simulink library "Lib_Solve_SSNRSolverJC_TMATS"  (R2015a)
settings: Solver=ode45  StartTime=0.0  StopTime=10.0  RelTol=1e-3
libraries: Lib_NM_JacobianCalc_TMATS x1, Lib_NM_NewtonRaphsonSolver_TMATS x1
Description:
  | Thomas Modules
settings Model: Creator=jwchapm2  LastModifiedBy=jwchapm2
settings OptimizationCC: ExpressionDepthLimit=2147483647
settings DebuggingCC: UnderspecifiedInitializationDetection=Classic  MergeDetectMultiDrivingBlocksExec=none  SolverPrmCheckMsg=warning  StateNameClashWarn=warning

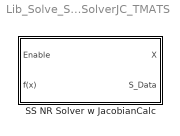
== system Lib_Solve_SSNRSolverJC_TMATS ==
  SS NR Solver w JacobianCalc : Subsystem  mask(T-MATS: SS NR Solver w Jacobian Calc Library Block){SJac_Per_M=[0.01 0.01 0.01;-0.01 -0.01,-0.01], SNR_IC_M=[1; 2; 3], SNR_DX_M=5, SNR_Mx_M=100000, SNR_Mn_M=0.00001, SJacobianAttempts_M=20, Cond_Limits_M=0.0001}
      mask prompts: SJac_Per_M "SJac_Per_M - Jacobian Perturbation size (frac)(nxm)"; SNR_IC_M "SNR_IC_M - Newton Raphson Initial Conditions (mx1)"; SNR_DX_M "SNR_DX_M - Newton Raphson step size limit (%) (1x1)"; SNR_Mx_M "SNR_Mx_M - Newton Raphson max limit (1x1 or mx1)"; SNR_Mn_M "SNR_Mn_M - Newton Raphson min limit (1x1 or mx1)"; SJacobianAttempts_M "SJacobianAttempts_M - Newton Raphson attempts before the Jacobian recalculation (1x1)"; Cond_Limits_M "Cond_Limits_M - Iteration Conditions Limits (mx1 or 1x1)"
      mask help:
      | The Steady State Newton Raphson Solver with Jacobian Calculator block will
      | supply the inputs to iteratively drive the outputs of a system to zero.
      |
      | This will be performed in three steps.
      | 1) Jabobian calculator sends Perturbations to the plant then calculates the plant
      | Jacboian based on the system response
      | 2) The Newton Raphson will use the inverse of the Jacobian to iteratively step the
      | system toward solution.
      | 3) Once the solution has satisfied the conditions the Newton Raphson is shut off.
      |
      | Simulation run time length should be selected as to give the Newton Raphson solver adequate time to develop a solution.
      mask init:
      | if isequal(size(SNR_Mx_M),size(SNR_IC_M))
      | elseif isequal(size(SNR_Mx_M),[1 1])
      | else
      |     disp('NR_Mx_Lim_M must be the same size as NR_IC_M or a constant')
      | end
      | 
      | if isequal(size(SNR_Mn_M),size(SNR_IC_M))
      | elseif isequal(size(SNR_Mn_M),[1 1])
      | else
      |     disp('NR_Mn_Lim_M must be the same size as NR_IC_M or a constant')
      | end
      mask Help: web(which('Solver_TMATS_SSNRwJC.html'),'-helpbrowser')

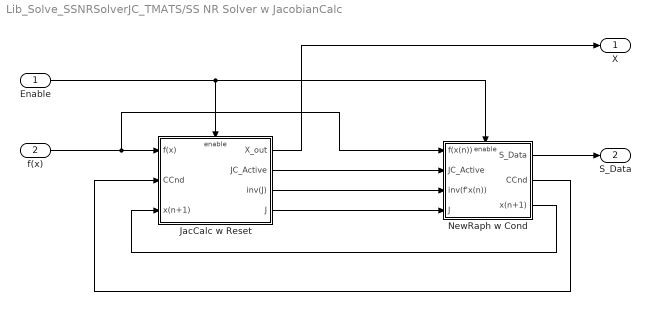
== system Lib_Solve_SSNRSolverJC_TMATS/SS NR Solver w JacobianCalc ==
  Enable : Inport  PortDimensions=1
  f(x) : Inport  Port=2  PortDimensions=length(SNR_IC_M)
  JacCalc w Reset : Subsystem  TreatAsAtomicUnit=on
  NewRaph w Cond : Subsystem  TreatAsAtomicUnit=on
  X : Outport  PortDimensions=length(SNR_IC_M)
  S_Data : Outport  Port=2  PortDimensions={1,[length(SNR_IC_M),length(SNR_IC_M)]}
  wires:
  JacCalc w Reset/1(X_out) -> X/1
  JacCalc w Reset/2(JC_Active) -> NewRaph w Cond/2(JC_Active)
  JacCalc w Reset/3(inv(J)) -> NewRaph w Cond/3(inv(f'x(n)))
  JacCalc w Reset/4(J) -> NewRaph w Cond/4(J)
  NewRaph w Cond/2(CCnd) -> JacCalc w Reset/2(CCnd)
  f(x)/1 -> NewRaph w Cond/1(f(x(n))), JacCalc w Reset/1(f(x))
  NewRaph w Cond/3(x(n+1)) -> JacCalc w Reset/3(x(n+1))
  NewRaph w Cond/1(S_Data) -> S_Data/1
  Enable/1 -> NewRaph w Cond/Enable, JacCalc w Reset/Enable

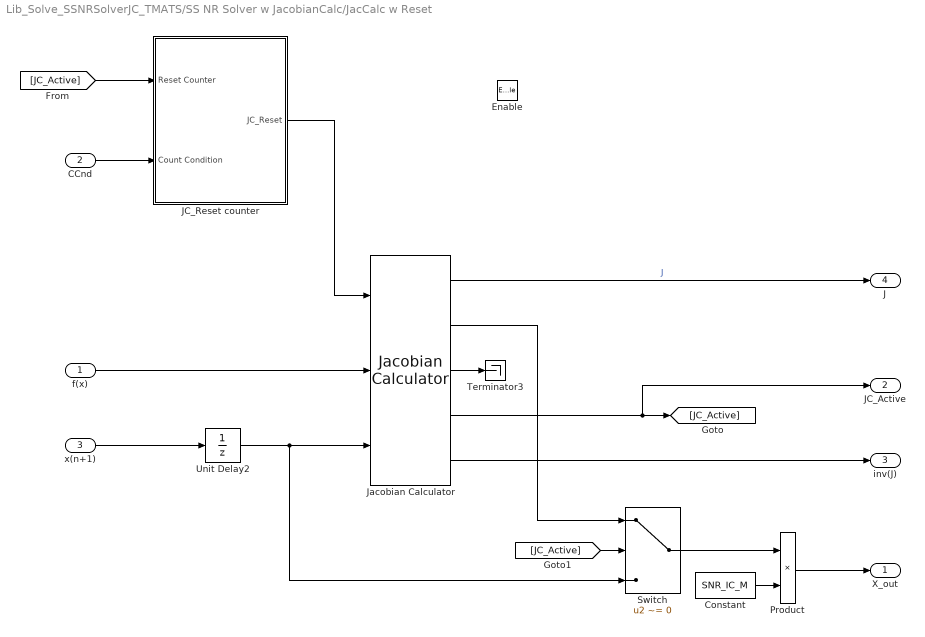
== system Lib_Solve_SSNRSolverJC_TMATS/SS NR Solver w JacobianCalc/JacCalc w Reset ==
  f(x) : Inport  PortDimensions=length(SNR_IC_M)
  CCnd : Inport  Port=2  PortDimensions=1
  x(n+1) : Inport  Port=3  PortDimensions=length(SNR_IC_M)
  Enable : EnablePort
  Constant : Constant  Value=SNR_IC_M
  JC_Reset counter : Subsystem
  Jacobian Calculator : Lib_NM_JacobianCalc_TMATS/Jacobian Calculator  N_Per_M=SJac_Per_M
  Product : Product  RndMeth=Zero
  Switch : Switch  Criteria=u2 ~= 0  Threshold=1
  Terminator3 : Terminator
  Unit Delay2 : UnitDelay  InitialCondition=ones(length(SNR_IC_M),1)  SampleTime=-1
  X_out : Outport  PortDimensions=length(SNR_IC_M)
  JC_Active : Outport  Port=2  PortDimensions=1
  inv(J) : Outport  Port=3  PortDimensions=[length(SNR_IC_M),length(SNR_IC_M)]
  J : Outport  Port=4  PortDimensions=[length(SNR_IC_M),length(SNR_IC_M)]
  wires:
  Jacobian Calculator/3 -> Terminator3/1
  Jacobian Calculator/2 -> Switch/1
  Jacobian Calculator/4 -> JC_Active/1, [JC_Active]
  Unit Delay2/1 -> Switch/3, Jacobian Calculator/3
  Constant/1 -> Product/2
  Jacobian Calculator/5 -> inv(J)/1
  [JC_Active] -> JC_Reset counter/1(Reset Counter)
  Switch/1 -> Product/1
  Jacobian Calculator/1 -> J/1  "J"
  Product/1 -> X_out/1
  JC_Reset counter/1(JC_Reset) -> Jacobian Calculator/1
  x(n+1)/1 -> Unit Delay2/1
  CCnd/1 -> JC_Reset counter/2(Count Condition)
  [JC_Active] -> Switch/2
  f(x)/1 -> Jacobian Calculator/2

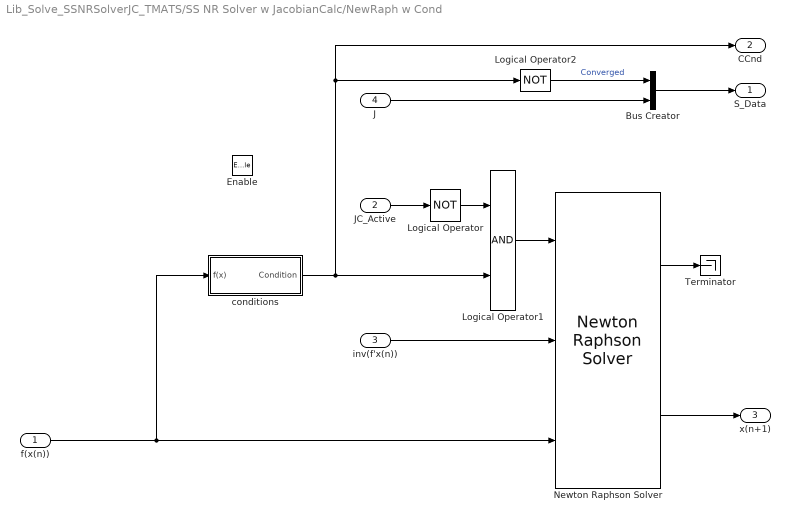
== system Lib_Solve_SSNRSolverJC_TMATS/SS NR Solver w JacobianCalc/NewRaph w Cond ==
  f(x(n)) : Inport  PortDimensions=length(SNR_IC_M)
  JC_Active : Inport  Port=2  PortDimensions=1
  inv(f'x(n)) : Inport  Port=3  PortDimensions=[length(SNR_IC_M),length(SNR_IC_M)]
  J : Inport  Port=4  PortDimensions=[length(SNR_IC_M), length(SNR_IC_M)]
  Enable : EnablePort
  Bus Creator : BusCreator  Inputs=2
  Logical Operator : Logic  Operator=NOT  AllPortsSameDT=off  OutDataTypeStr=boolean
  Logical Operator1 : Logic  AllPortsSameDT=off  OutDataTypeStr=boolean
  Logical Operator2 : Logic  Operator=NOT  AllPortsSameDT=off  OutDataTypeStr=boolean
  Newton Raphson Solver : Lib_NM_NewtonRaphsonSolver_TMATS/Newton Raphson Solver  NR_IC_M=ones(size(SNR_IC_M))  NR_dx_Lim_M=SNR_DX_M  NR_Mx_Lim_M=SNR_Mx_M./SNR_IC_M  NR_Mn_Lim_M=SNR_Mn_M./SNR_IC_M  BlkNm_M=double(gcb)
  Terminator : Terminator
  conditions : Subsystem
  S_Data : Outport  PortDimensions={1,[length(SNR_IC_M),length(SNR_IC_M)]}
  CCnd : Outport  Port=2  PortDimensions=1
  x(n+1) : Outport  Port=3  PortDimensions=length(SNR_IC_M)
  wires:
  Bus Creator/1 -> S_Data/1
  Logical Operator/1 -> Logical Operator1/1
  Logical Operator1/1 -> Newton Raphson Solver/1
  conditions/1(Condition) -> Logical Operator2/1, CCnd/1, Logical Operator1/2
  Logical Operator2/1 -> Bus Creator/1  "Converged"
  JC_Active/1 -> Logical Operator/1
  inv(f'x(n))/1 -> Newton Raphson Solver/2
  Newton Raphson Solver/1 -> Terminator/1
  Newton Raphson Solver/2 -> x(n+1)/1
  J/1 -> Bus Creator/2
  f(x(n))/1 -> conditions/1(f(x)), Newton Raphson Solver/3

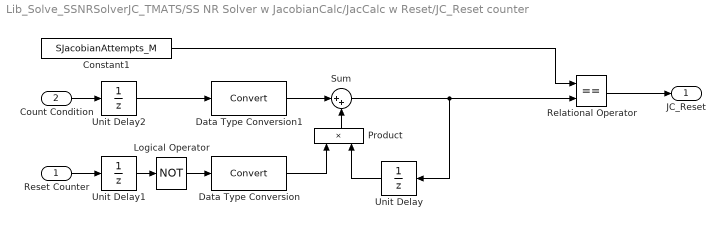
== system Lib_Solve_SSNRSolverJC_TMATS/SS NR Solver w JacobianCalc/JacCalc w Reset/JC_Reset counter ==
  Reset Counter : Inport
  Count Condition : Inport  Port=2
  Constant1 : Constant  Value=SJacobianAttempts_M
  Data Type Conversion : DataTypeConversion
  Data Type Conversion1 : DataTypeConversion
  Logical Operator : Logic  Operator=NOT  AllPortsSameDT=off  OutDataTypeStr=boolean
  Product : Product  RndMeth=Zero
  Relational Operator : RelationalOperator  Operator===  OutDataTypeStr=boolean
  Sum : Sum  Inputs=|++
  Unit Delay : UnitDelay  SampleTime=-1
  Unit Delay1 : UnitDelay  SampleTime=-1
  Unit Delay2 : UnitDelay  SampleTime=-1
  JC_Reset : Outport
  wires:
  Constant1/1 -> Relational Operator/1
  Relational Operator/1 -> JC_Reset/1
  Product/1 -> Sum/2
  Reset Counter/1 -> Unit Delay1/1
  Unit Delay/1 -> Product/2
  Data Type Conversion/1 -> Product/1
  Data Type Conversion1/1 -> Sum/1
  Unit Delay1/1 -> Logical Operator/1
  Logical Operator/1 -> Data Type Conversion/1
  Count Condition/1 -> Unit Delay2/1
  Unit Delay2/1 -> Data Type Conversion1/1
  Sum/1 -> Unit Delay/1, Relational Operator/2

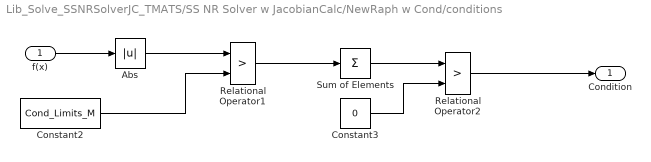
== system Lib_Solve_SSNRSolverJC_TMATS/SS NR Solver w JacobianCalc/NewRaph w Cond/conditions ==
  f(x) : Inport
  Abs : Abs
  Constant2 : Constant  Value=Cond_Limits_M
  Constant3 : Constant  Value=0
  Relational Operator1 : RelationalOperator  Operator=>  OutDataTypeStr=boolean
  Relational Operator2 : RelationalOperator  Operator=>  OutDataTypeStr=boolean
  Sum of Elements : Sum  Inputs=+
  Condition : Outport
  wires:
  Constant2/1 -> Relational Operator1/2
  Relational Operator1/1 -> Sum of Elements/1
  Constant3/1 -> Relational Operator2/2
  Abs/1 -> Relational Operator1/1
  Sum of Elements/1 -> Relational Operator2/1
  f(x)/1 -> Abs/1
  Relational Operator2/1 -> Condition/1
